simulink model "airTrackLab"  (R2021a)
settings: Solver=ode23t  StartTime=0.0  StopTime=30  FixedStep=0.02  MaxStep=0.01  RelTol=1e-3  AbsTol=1e-4  EnableMultiTasking=on
PostLoadFcn:
  | disp('default settings')
  | 
  | % Default starting positions
  | x0_cart1 = -0.2
  | x0_cart2 = 0.8
  | x0_gate1 = -0.4
  | x0_gate2 = 0.4
  | 
  | % How much damping the carts feel
  | dampingCoef = 0.01 % N/(m/s)
  | 
  | % Hanger damping
  | pulleyDamping = 0;
  | 
  | % Max measurement noise for the gates
  | noise_max = 0.01 % seconds
  | 
  | % How many time steps to show in the history
  | nHistory = 4
  | 
  | % Based on the provided STLs
  | cart_length = 0.15
  | 
  | subsystems = find_system(gcs,'BlockType','SubSystem');
  | p = Simulink.Mask.get(subsystems{1});
  | p.Parameters(1).Value = '-0.8';
  | p.Parameters(2).Value = '0';
  | p.Parameters(3).Value = '-0.4';
  | p.Parameters(4).Value = '0.4';
  | p.Parameters(5).Value = '0';
  | p.Parameters(6).Value = '0';
  | 
  | % Resize the model window
  | set(0,"Units","pixels")
  | sSize = get(0,"screensize");
  | set_param(gcs,'location',...
  |     [1,sSize(4)*0.01,round(sSize(3)/2),sSize(4)*0.96]);
  | 
  | % Reset the zoom
  | set_param(gcs, 'ZoomFactor','FitSystem')
undefined symbols (not defined in the file): X, Y, Z
libraries: sm_lib x104, simulink x12, nesl_utility x9
(part 1 of 3)
settings Model: EnablePacing=on  OrderedModelArguments=off  Creator=Rocksmithed  LastModifiedBy=Work
settings SolverCC: AutoScaleAbsTol=off  AlgebraicLoopSolver=TrustRegion
settings DataIOCC: LimitDataPoints=on  MaxDataPoints=10000
settings OptimizationCC: LifeSpan=inf
settings DebuggingCC: AllowSymbolicDim=off  SFUnexpectedBacktrackingDiag=warning  SFNoUnconditionalDefaultTransitionDiag=warning  SFExecutionAtInitializationDiag=none  SFMachineParentedDataDiag=warning  ArithmeticOperatorsInVariantConditions=warning
settings SFSimCC: SimUseLocalCustomCode=off  CustomCodeUndefinedFunction=UseInterfaceOnly
settings RTWCC: RTWUseLocalCustomCode=off
settings CodeAppCC: StateflowObjectComments=on
settings GRTTargetCC: TargetLangStandard=C89/C90 (ANSI)
settings ConfigComp: CovMetricSettings=dw  CovSaveCumulativeToWorkspaceVar=on  CovSaveSingleToWorkspaceVar=on  CovExternalEMLEnable=off  CovSFcnEnable=off
settings SimscapeCC: SimscapeLogType=all  SimscapeLogSimulationStatistics=on  SimscapeLogDataHistory=10000
settings ExplorerConfigSet: InternalSimMechanicsExplorerSettings="<ExplorerConfiguration><canonicalview>default</canonicalview><AnimationSetting><BasePlaybackSpeed>1.0</BasePlaybackSpeed><PlaybackSpeedFactor>1.0</PlaybackSpeedFactor></AnimationSetting><TilePanel><TileInfo><Tiles Columns=\"2\" Count=\"3\" Rows=\"2\"><Column Weight=\"0.8233\"/><Column Weight=\"0.1767\"/><Row Weight=\"0.2309\"/><Row Weight=\"0.7691\"/><Tile Height=\"1\" Width=\"2\" X=\"0\" Y=\"0\"/><Tile Height=\"1\" Width=\"1\" X=\"0\" Y=\"1\"/><Tile Height=\"1\" Width=\"1\" X=\"1\" Y=\"1\"/></Tiles></TileInfo><SceneInfo><SceneViewer><BGColor><R>1</R><G>1</G><B>1</B></BGColor><Camera><DoPerspective>off</DoPerspective><Position><X>0.018300882451578071</X><Y>-1.66502198042091809</Y><Z>0.155363278025413054</Z></Position><Center><X>0.018300882451578071</X><Y>9.39015043499580315e-09</Y><Z>0.155363278025413054</Z></Center><Up><X>0</X><Y>-0</Y><Z>1</Z></Up><ViewLimDist>1</ViewLimDist><YLim>0.387195273745834012</YLim><XLim>1.19850444036210479</XLim></Camera></SceneViewer><SceneViewer><BGColor><R>1</R><G>1</G><B>1</B></BGColor><Camera><DoPerspective>off</DoPerspective><Position><X>1.92657717822519481</X><Y>-0.555217561550410799</Y><Z>0.43190835445211162</Z></Position><Center><X>0.000630036713113105943</X><Y>-0.00292388052674194803</Y><Z>0.127558358447527082</Z></Center><Up><X>-0.139841397017632707</X><Y>0.0570909199469538109</Y><Z>0.988526686812130406</Z></Up><ViewLimDist>1</ViewLimDist><YLim>0.492618300070346571</YLim><XLim>0.372709129942266348</XLim></Camera></SceneViewer><SceneViewer><BGColor><R>1</R><G>1</G><B>1</B></BGColor><Camera><DoPerspective>off</DoPerspective><Position><X>1.02205702851478053</X><Y>-1.66502198042091809</Y><Z>-0.681352306661953344</Z></Position><Center><X>1.02205702851478053</X><Y>8.09732611517510747e-09</Y><Z>-0.681352306661953344</Z></Center><Up><X>0</X><Y>-0</Y><Z>1</Z></Up><ViewLimDist>1</ViewLimDist><YLim>1.06828991799173401</YLim><XLim>0.17113382181420983</XLim></Camera></SceneViewer></SceneInfo></TilePanel><MechEditorPanel><Cameras><Camera><Id>Camera1</Id><Value><Name>Camera1</Name><NativeCamera><PositionKeyframeSet><Keyframe><Time>30</Time><Value><X>-0.06353733975693017</X><Y>-1.5549717096079039</Y><Z>0.94456927641812571</Z></Value></Keyframe></PositionKeyframeSet><CenterKeyframeSet><Keyframe><Time>30</Time><Value><X>-0.014695794825631658</X><Y>-0.017005502884078094</Y><Z>0.19960924384738066</Z></Value></Keyframe></CenterKeyframeSet><UpVectorKeyframeSet><Keyframe><Time>30</Time><Value><X>-0.0033381063490633966</X><Y>0.43601551279510337</Y><Z>0.89993295841858445</Z></Value></Keyframe></UpVectorKeyframeSet></NativeCamera></Value></Camera></Cameras><GfxPanelCameraMap/><VideoCreator><PlaybackSpeedRatio>1.0</PlaybackSpeedRatio><FrameRate>30</FrameRate><VideoFormat>Motion JPEG AVI</VideoFormat><FrameSize>auto</FrameSize></VideoCreator></MechEditorPanel></ExplorerConfiguration>"

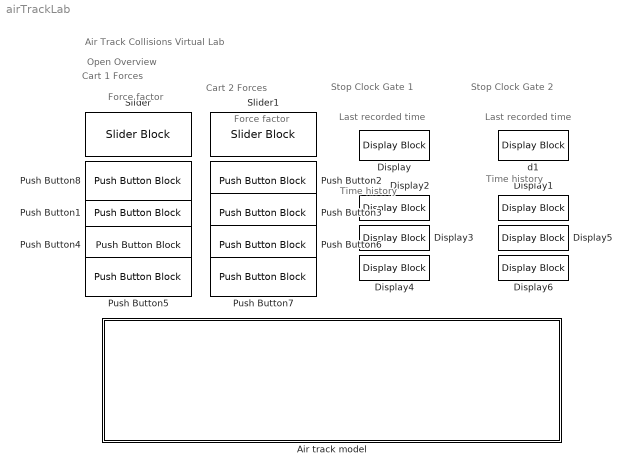
== system airTrackLab ==
  note: Air Track Collisions Virtual Lab
  note: Open Overview
  note: Force factor
  note: Stop Clock Gate 2
  note: Cart 1 Forces
  note: Cart 2 Forces
  note: Stop Clock Gate 1
  note: Force factor
  note: Last recorded time
  note: Time history
  note: Last recorded time
  note: Time history
  Air track model : Subsystem  InitFcn=|  mask{popup_collisionType=Elastic, x0_cart1=-0.8, x0_gate1=-0.4, x0_cart2=0, x0_gate2=0.4, popup_extraMassC1=0 plates (0 g), popup_extraMassC2=0 plates (0 g), popup_hangingMass=0 plates (0 g)}
      | if(x0_cart1 > x0_cart2)
      | 	error('Set cart 2 to be on the + side of cart 1')
      |    x0_cart1 = -0.75;
      |    x0_cart2 = 0.75;
      | end
      mask prompts: popup_collisionType "Collisions"; x0_cart1 "Cart 1 x0 [m] (must be left of Cart 2)"; x0_gate1 "Gate 1 x [m]"; x0_cart2 "Cart 2 x0 [m] (must be right of Cart 1)"; x0_gate2 "Gate 2 x [m]"; popup_extraMassC1 "Cart 1"; popup_extraMassC2 "Cart 2"; popup_hangingMass "Hanging"
      mask init:
      | set_param([gcb '/Contact Force'],'LabelModeActiveChoice',get_param(gcb,'popup_collisionType'));
      | switch(get_param(gcb,'popup_extraMassC1'))
      |     case '0 plates (0 g)', vntstrC1 = 'None';
      |     case '1 plate (100 g)', vntstrC1 = 'Plates_1';
      |     case '2 plates (200 g)',vntstrC1 = 'Plates_2';
      |     case '3 plates (300 g)',vntstrC1 = 'Plates_3';
      | end
      | set_param([gcb '/Mass Cart 1'],'LabelModeActiveChoice',vntstrC1);
      | switch(get_param(gcb,'popup_extraMassC2'))
      |     case '0 plates (0 g)', vntstrC2 = 'None';
      |     case '1 plate (100 g)', vntstrC2 = 'Plates_1';
      |     case '2 plates (200 g)',vntstrC2 = 'Plates_2';
      |     case '3 plates (300 g)',vntstrC2 = 'Plates_3';
      | end
      | set_param([gcb '/Mass Cart 2'],'LabelModeActiveChoice',vntstrC2);
      | 
      | switch(get_param(gcb,'popup_hangingMass'))
      |     case '0 plates (0 g)', vntstrH = 'None'; 
      |     case '1 plate (100 g)', vntstrH = 'Plates_1';
      |     case '2 plates (200 g)',vntstrH = 'Plates_2';
      |     case '3 plates (300 g)',vntstrH = 'Plates_3';
      | end
      | if(strcmp(vntstrH,'None'))
      | set_param([gcb '/Load'],'LabelModeActiveChoice','None');
      | else
      | set_param([gcb '/Load'],'LabelModeActiveChoice','Hanging_Mass');
      | set_param([gcb '/Load/Hanging Mass/Mass'],'LabelModeActiveChoice',vntstrH);
      | end
      mask TypeOptions popup_collisionType: Elastic | Inelastic
      mask Callback x0_cart1:
      | maskObj = Simulink.Mask.get(gcb);
      | x0c1_h = maskObj.getParameter('x0_cart1');
      | x0c2_h = maskObj.getParameter('x0_cart2');
      | if(str2num(x0c2_h.Value)<=(str2num(x0c1_h.Value)+0.165))
      |    x0c2_h.Value=num2str(round(str2num(x0c1_h.Value)+0.165+0.0005,3));
      |    %x0c2_h.Value = num2str(0);
      | end
      | x0c2_h.Range=[str2num(x0c1_h.Value)+0.165 0.8];
      | 
      | %clear maskObj
      mask Callback x0_cart2:
      | maskObj = Simulink.Mask.get(gcb);
      | x0c1_h = maskObj.getParameter('x0_cart1');
      | x0c2_h = maskObj.getParameter('x0_cart2');
      | if(str2num(x0c1_h.Value)>=(str2num(x0c2_h.Value)-0.165))
      |    x0c2_h.Value=num2str(round(str2num(x0c2_h.Value)-0.165-0.0005,3));
      |    %x0c2_h.Value = num2str(0);
      | end
      | x0c1_h.Range=[-0.8 str2num(x0c2_h.Value)-0.165];
      mask TypeOptions popup_extraMassC1: 0 plates (0 g) | 1 plate (100 g) | 2 plates (200 g) | 3 plates (300 g)
      mask TypeOptions popup_extraMassC2: 0 plates (0 g) | 1 plate (100 g) | 2 plates (200 g) | 3 plates (300 g)
      mask TypeOptions popup_hangingMass: 0 plates (0 g) | 1 plate (100 g) | 2 plates (200 g) | 3 plates (300 g)
      mask DialogControl Container7 Prompt: Experiments
      mask DialogControl push_default Prompt: Default Setup
      mask DialogControl push_default Callback:
      | maskObj = Simulink.Mask.get(gcb);
      | x0c1_h = maskObj.getParameter('x0_cart1');
      | x0c1_h.Value = '-0.8';
      | x0c2_h = maskObj.getParameter('x0_cart2');
      | x0c2_h.Value = '0';
      | 
      | x0c1_h.Range = [-0.8 -0.165];
      | x0c2_h.Range = [-0.635 0.8];
      | 
      | x0g1_h = maskObj.getParameter('x0_gate1');
      | x0g1_h.Value = '-0.4';
      | x0g2_h = maskObj.getParameter('x0_gate2');
      | x0g2_h.Value = '0.4';
      | pmc1_h = maskObj.getParameter('popup_extraMassC1');
      | pmc1_h.Value = '0 plates (0 g)';
      | pmc2_h = maskObj.getParameter('popup_extraMassC2');
      | pmc2_h.Value = '0 plates (0 g)';
      | phm_h = maskObj.getParameter('popup_hangingMass');
      | phm_h.Value = '0 plates (0 g)';
      | pct_h = maskObj.getParameter('popup_collisionType');
      | pct_h.Value = 'Elastic';
      | 
      | clear maskObj
      mask DialogControl push_default_copy Prompt: 1. Elastic
      mask DialogControl push_default_copy Callback:
      | maskObj = Simulink.Mask.get(gcb);
      | x0c1_h = maskObj.getParameter('x0_cart1');
      | x0c1_h.Value = '-0.8';
      | x0c2_h = maskObj.getParameter('x0_cart2');
      | x0c2_h.Value = '0';
      | 
      | x0c1_h.Range = [-0.8 -0.165];
      | x0c2_h.Range = [-0.635 0.8];
      | 
      | x0g1_h = maskObj.getParameter('x0_gate1');
      | x0g1_h.Value = '-0.4';
      | x0g2_h = maskObj.getParameter('x0_gate2');
      | x0g2_h.Value = '0.4';
      | pmc1_h = maskObj.getParameter('popup_extraMassC1');
      | pmc1_h.Value = '0 plates (0 g)';
      | pmc2_h = maskObj.getParameter('popup_extraMassC2');
      | pmc2_h.Value = '0 plates (0 g)';
      | phm_h = maskObj.getParameter('popup_hangingMass');
      | phm_h.Value = '0 plates (0 g)';
      | pct_h = maskObj.getParameter('popup_collisionType');
      | pct_h.Value = 'Elastic';
      | 
      | clear maskObj
      mask DialogControl push_default_copy_copy Prompt: 2. Inelastic
      mask DialogControl push_default_copy_copy Callback:
      | maskObj = Simulink.Mask.get(gcb);
      | x0c1_h = maskObj.getParameter('x0_cart1');
      | x0c1_h.Value = '-0.8';
      | x0c2_h = maskObj.getParameter('x0_cart2');
      | x0c2_h.Value = '0';
      | 
      | x0c1_h.Range = [-0.8 -0.165];
      | x0c2_h.Range = [-0.635 0.8];
      | 
      | x0g1_h = maskObj.getParameter('x0_gate1');
      | x0g1_h.Value = '-0.4';
      | x0g2_h = maskObj.getParameter('x0_gate2');
      | x0g2_h.Value = '0.4';
      | pmc1_h = maskObj.getParameter('popup_extraMassC1');
      | pmc1_h.Value = '3 plates (300 g)';
      | pmc2_h = maskObj.getParameter('popup_extraMassC2');
      | pmc2_h.Value = '0 plates (0 g)';
      | phm_h = maskObj.getParameter('popup_hangingMass');
      | phm_h.Value = '0 plates (0 g)';
      | pct_h = maskObj.getParameter('popup_collisionType');
      | pct_h.Value = 'Inelastic';
      | 
      | clear maskObj
      mask DialogControl push_default_copy_copy_copy Prompt: 3. Energy
      mask DialogControl push_default_copy_copy_copy Callback:
      | maskObj = Simulink.Mask.get(gcb);
      | x0c1_h = maskObj.getParameter('x0_cart1');
      | x0c1_h.Value = '-0.8';
      | x0c2_h = maskObj.getParameter('x0_cart2');
      | x0c2_h.Value = '0';
      | 
      | x0c1_h.Range = [-0.8 -0.165];
      | x0c2_h.Range = [-0.635 0.8];
      | 
      | x0g1_h = maskObj.getParameter('x0_gate1');
      | x0g1_h.Value = '0.3';
      | x0g2_h = maskObj.getParameter('x0_gate2');
      | x0g2_h.Value = '0.6';
      | pmc1_h = maskObj.getParameter('popup_extraMassC1');
      | pmc1_h.Value = '0 plates (0 g)';
      | pmc2_h = maskObj.getParameter('popup_extraMassC2');
      | pmc2_h.Value = '2 plates (200 g)';
      | phm_h = maskObj.getParameter('popup_hangingMass');
      | phm_h.Value = '1 plate (100 g)';
      | pct_h = maskObj.getParameter('popup_collisionType');
      | pct_h.Value = 'Elastic';
      | 
      | clear maskObj
      mask DialogControl Container10 Prompt: Extra Mass
      mask Display:
      | image('airTrackMask.png','center');
      | text(0.12, 0.79, 'Cart 1', 'horizontalAlignment', 'center')
      | text(0.86, 0.79, 'Cart 2', 'horizontalAlignment', 'center')
      | 
      | text(0.32, 0.87, 'Gate 1', 'horizontalAlignment', 'center')
      | text(0.67, 0.87, 'Gate 2', 'horizontalAlignment', 'center')
      | 
      | text(0.5, 0.1, 'Double-click here to set starting positions and weights', 'horizontalAlignment', 'center')
      | 
      | text(0.91, 0.17, '+ direction', 'horizontalAlignment', 'center')
  Display{,1..4} (5 alike) : DisplayBlock  LabelPosition=Hide  Format=short  Transparency=1
  Display5 : DisplayBlock  LabelPosition=Hide  Format=short  Transparency=1  Layout=Fill available space
  Display6 : DisplayBlock  LabelPosition=Hide  Format=short  Transparency=1  Layout=Fill available space
  Push Button1 : PushButtonBlock  ButtonText=Apply force -x
  Push Button2 : PushButtonBlock  ButtonText=Apply force +x
  Push Button3 : PushButtonBlock  ButtonText=Apply force -x
  Push Button4 : PushButtonBlock  ButtonText=Pulse +x (0.1 sec)
  Push Button5 : PushButtonBlock  ButtonText=Pulse -x (0.1 sec)  OnValue=-1
  Push Button6 : PushButtonBlock  ButtonText=Pulse +x (0.1 sec)
  Push Button7 : PushButtonBlock  ButtonText=Pulse -x (0.1 sec)  OnValue=-1
  Push Button8 : PushButtonBlock  ButtonText=Apply force +x
  Slider : SliderBlock  LabelPosition=Hide  ScaleMax=1  TickInterval=0.25
  Slider1 : SliderBlock  LabelPosition=Hide  ScaleMax=1  TickInterval=0.25
  d1 : DisplayBlock  LabelPosition=Hide  Format=short  Transparency=1  Layout=Fill available space

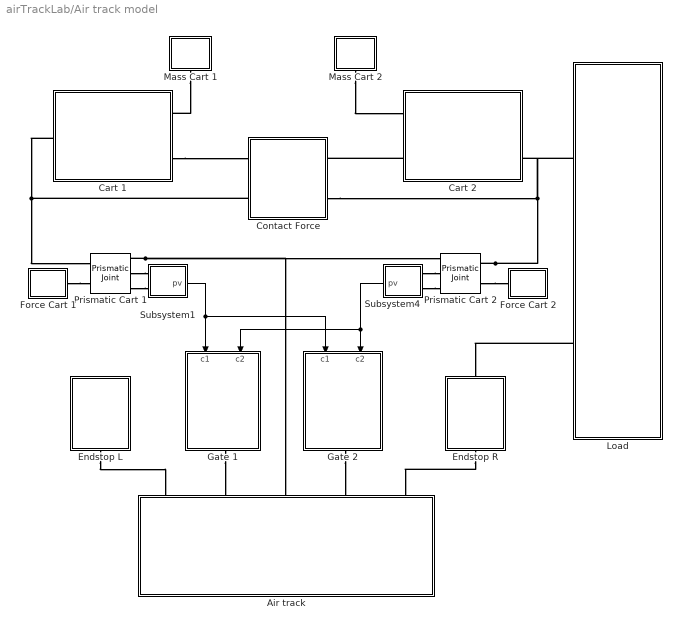
== system airTrackLab/Air track model ==
  Air track : Subsystem
      settings: PortSchema="{\"entries\":[{\"content\":{\"sides\":[{\"content\":{\"connectorIds\":[]},\"type\":\"ConnectorPlacement.EquallySpacedRectSide\",\"uuid\":\"090b3a62-51f7-462c-98c5-a584c300c54a\"},{\"content\":{\"connectorIds\":[],\"side\":\"RIGHT\"},\"type\":\"ConnectorPlacement.EquallySpacedRectSide\",\"uuid\":\"a4dd45ef-3830-4d80-a6d2-012ce92ee2ce\"},{\"content\":{\"connectorIds\":[],\"side\":\"TOP\"},\"type\":\"ConnectorPlacement.EquallySpacedRectSide\",\"uuid\":\"395c260b-744a-480a-9e83-719a01711115\"},{\"content\":{\"connectorIds\":[\"RConn1\",\"RConn2\",\"RConn3\",\"RConn4\",\"RConn5\"],\"side\":\"BOTTOM\"},\"type\":\"ConnectorPlacement.EquallySpacedRectSide\",\"uuid\":\"a18b275a-4662-4f32-9408-960fb193559a\"}]},\"type\":\"ConnectorPlacement.EquallySpacedConnector\",\"uuid\":\"2f11ba3c-3a56-4e43-8d79-c5dc35ee6124\"}],\"packageUris\":[\"http://schema.mathworks.com/mf0/Connector/R2020b\"],\"version\":\"1.0\"}"
      mask Display: image('airTrack.png');
  Cart 1 : Subsystem
      mask Display: image('cart.png');
  Cart 2 : Subsystem
      mask Display: image('cart.png');
  Contact Force : Subsystem  Variant=on  VariantControlMode=label  VariantControl=Choice  LabelModeActiveChoice=Elastic
  Endstop L : Subsystem
      mask Display: image('stop.png');
  Endstop R : Subsystem
      mask Display: image('stop.png');
  Force Cart 1 : Subsystem
  Force Cart 2 : Subsystem
  Gate 1 : Subsystem
      mask Display: image('gate1.png');
  Gate 2 : Subsystem
      mask Display: image('gate2.png');
  Load : Subsystem  Variant=on  VariantControlMode=label  VariantControl=Choice  LabelModeActiveChoice=None
      settings: AttributesFormatString=%<LabelModeActiveChoice>
  Mass Cart 1 : Subsystem  Variant=on  VariantControlMode=label  VariantControl=Choice  LabelModeActiveChoice=None
      settings: AttributesFormatString=%<LabelModeActiveChoice>
  Mass Cart 2 : Subsystem  Variant=on  VariantControlMode=label  VariantControl=Choice  LabelModeActiveChoice=None
      settings: AttributesFormatString=%<LabelModeActiveChoice>
  Prismatic Cart 1 : sm_lib/Joints/Prismatic Joint  JointMode=Normal  SenseConstraintForce=off  SenseConstraintForceX=off  SenseConstraintForceY=off  SenseConstraintForceZ=off  SenseConstraintTorque=off  SenseConstraintTorqueX=off  SenseConstraintTorqueY=off  SenseConstraintTorqueZ=off  SenseTotalForce=off  SenseTotalForceX=off  SenseTotalForceY=off  SenseTotalForceZ=off  SenseTotalTorque=off  SenseTotalTorqueX=off  SenseTotalTorqueY=off  SenseTotalTorqueZ=off  CompositeWrenchDir=FollowerOnBase  CompositeWrenchFrame=BaseFrame  EquilibriumPosition=0  EquilibriumPositionUnits=m  SpringStiffness=0  SpringStiffnessUnits=N/m  DampingCoefficient=dampingCoef  DampingCoefficientUnits=N/(m/s)  TorqueActuationMode=InputTorque  MotionActuationMode=ComputedMotion  SensePosition=on  SenseVelocity=on  SenseAcceleration=off  SenseTorqueForce=off  SenseLowerLimitTorqueForce=off  SenseUpperLimitTorqueForce=off  LowerLimitSpecify=on  LowerLimitBound=-0.9  LowerLimitBoundUnits=m  LowerLimitStiffness=1e9  LowerLimitStiffnessUnits=N/m  LowerLimitDamping=0.1  LowerLimitDampingUnits=N/(m/s)  LowerLimitTransitionRegionWidth=1e-4  LowerLimitTransitionRegionWidthUnits=m  UpperLimitSpecify=on  UpperLimitBound=0.9  UpperLimitBoundUnits=m  UpperLimitStiffness=1e9  UpperLimitStiffnessUnits=N/m  UpperLimitDamping=0.1  UpperLimitDampingUnits=N/(m/s)  UpperLimitTransitionRegionWidth=1e-4  UpperLimitTransitionRegionWidthUnits=m  PositionTargetSpecify=on  PositionTargetPriority=High  PositionTargetValue=x0_cart1  PositionTargetValueUnits=m  VelocityTargetSpecify=off  VelocityTargetPriority=High  VelocityTargetValue=0.5  VelocityTargetValueUnits=m/s
  Prismatic Cart 2 : sm_lib/Joints/Prismatic Joint  JointMode=Normal  SenseConstraintForce=off  SenseConstraintForceX=off  SenseConstraintForceY=off  SenseConstraintForceZ=off  SenseConstraintTorque=off  SenseConstraintTorqueX=off  SenseConstraintTorqueY=off  SenseConstraintTorqueZ=off  SenseTotalForce=off  SenseTotalForceX=off  SenseTotalForceY=off  SenseTotalForceZ=off  SenseTotalTorque=off  SenseTotalTorqueX=off  SenseTotalTorqueY=off  SenseTotalTorqueZ=off  CompositeWrenchDir=FollowerOnBase  CompositeWrenchFrame=BaseFrame  EquilibriumPosition=0  EquilibriumPositionUnits=m  SpringStiffness=0  SpringStiffnessUnits=N/m  DampingCoefficient=dampingCoef  DampingCoefficientUnits=N/(m/s)  TorqueActuationMode=InputTorque  MotionActuationMode=ComputedMotion  SensePosition=on  SenseVelocity=on  SenseAcceleration=off  SenseTorqueForce=off  SenseLowerLimitTorqueForce=off  SenseUpperLimitTorqueForce=off  LowerLimitSpecify=on  LowerLimitBound=-0.9  LowerLimitBoundUnits=m  LowerLimitStiffness=1e9  LowerLimitStiffnessUnits=N/m  LowerLimitDamping=0.1  LowerLimitDampingUnits=N/(m/s)  LowerLimitTransitionRegionWidth=1e-4  LowerLimitTransitionRegionWidthUnits=m  UpperLimitSpecify=on  UpperLimitBound=0.9  UpperLimitBoundUnits=m  UpperLimitStiffness=1e9  UpperLimitStiffnessUnits=N/m  UpperLimitDamping=0.1  UpperLimitDampingUnits=N/(m/s)  UpperLimitTransitionRegionWidth=1e-4  UpperLimitTransitionRegionWidthUnits=m  PositionTargetSpecify=on  PositionTargetPriority=High  PositionTargetValue=x0_cart2  PositionTargetValueUnits=m  VelocityTargetSpecify=off  VelocityTargetPriority=High  VelocityTargetValue=0.5  VelocityTargetValueUnits=m/s
  Subsystem1 : Subsystem
  Subsystem4 : Subsystem
  wires:
  Subsystem1/1(pv) -> Gate 2/1(c1), Gate 1/1(c1)
  Subsystem4/1(pv) -> Gate 1/2(c2), Gate 2/2(c2)
  connections:
  Gate 2/RConn1 -- Air track/RConn2
  Gate 1/RConn1 -- Air track/RConn4
  Endstop L/RConn1 -- Air track/RConn5
  Endstop R/RConn1 -- Air track/RConn1
  Prismatic Cart 1/RConn3 -- Subsystem1/LConn2
  Prismatic Cart 1/RConn2 -- Subsystem1/LConn1
  Force Cart 1/RConn1 -- Prismatic Cart 1/LConn2
  Cart 1/RConn2 -- Contact Force/LConn1
  Subsystem4/LConn2 -- Prismatic Cart 2/RConn3
  Subsystem4/LConn1 -- Prismatic Cart 2/RConn2
  Prismatic Cart 2/LConn2 -- Force Cart 2/RConn1
  Prismatic Cart 1/RConn1 -- Prismatic Cart 2/RConn1 -- Air track/RConn3
  Mass Cart 2/RConn1 -- Cart 2/LConn1
  Cart 2/LConn2 -- Contact Force/RConn1
  Cart 1/LConn1 -- Prismatic Cart 1/LConn1 -- Contact Force/LConn2
  Prismatic Cart 2/LConn1 -- Contact Force/RConn2 -- Load/LConn1 -- Cart 2/RConn2
  Load/LConn2 -- Endstop R/LConn1
  Mass Cart 1/RConn1 -- Cart 1/RConn1

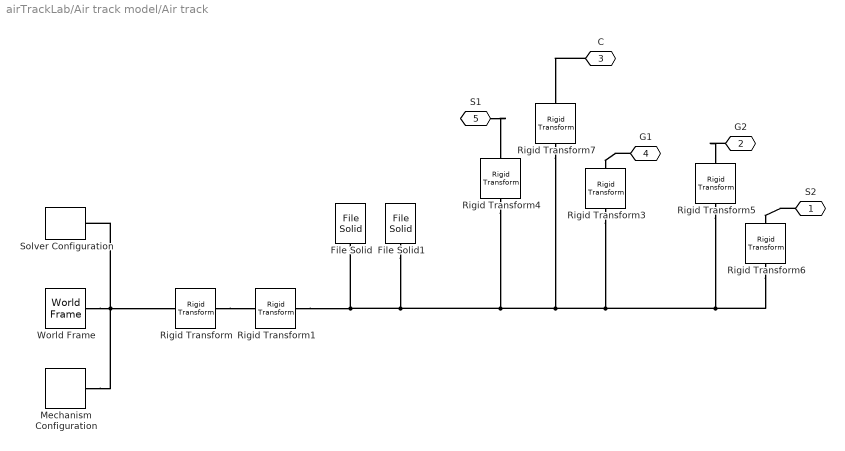
== system airTrackLab/Air track model/Air track ==
  File Solid : sm_lib/Body Elements/File Solid  ExtGeomFileName=airTrack.stl  UnitType=Custom  ExtGeomFileUnits=mm  StepReaderType=HEX  ExportConvexHullGeometry=off  InertiaType=CalculateFromGeometry  Mass=1  MassUnits=kg  CenterOfMass=[0 0 0]  CenterOfMassUnits=m  MomentsOfInertia=[1 1 1]  MomentsOfInertiaUnits=kg*m^2  ProductsOfInertia=[0 0 0]  ProductsOfInertiaUnits=kg*m^2  BasedOnType=Density  Density=1000  DensityUnits=kg/m^3  DoExposeReferenceFrame=on  SerializedFrames=<Frames><Frame><Id>Frame1</Id><Value><Name>F1</Name><Origin><Source>CenterOfMassFrame</Source><FeatureName></FeatureName></Origin><PrimaryAxis><DefinedDirection>+X</DefinedDirection><Source>ReferenceFrame</Source><SourceDirection>+Z</SourceDirection><FeatureName></FeatureName></PrimaryAxis><SecondaryAxis><DefinedDirection>+Y</DefinedDirection><Source>ReferenceFrame</Source><SourceDirection>+X</SourceDirection><FeatureName></FeatureName></SecondaryAxis></Value></Frame></Frames>  GraphicType=FromGeometry  MarkerShape=Sphere  MarkerSize=10  GraphicVisPropType=AdvancedVisualProperties  GraphicDiffuseColor=[0.8 0.8 0.81]  GraphicSpecularColor=[0.7 0.7 0.7 1]  GraphicAmbientColor=[0.05 0.05 0.05 1]  GraphicEmissiveColor=[0.05 0.05 0.05 1.0]  GraphicShininess=15  GraphicOpacity=1.0
  File Solid1 : sm_lib/Body Elements/File Solid  ExtGeomFileName=ruler.stl  UnitType=Custom  ExtGeomFileUnits=mm  StepReaderType=HEX  ExportConvexHullGeometry=off  InertiaType=CalculateFromGeometry  Mass=1  MassUnits=kg  CenterOfMass=[0 0 0]  CenterOfMassUnits=m  MomentsOfInertia=[1 1 1]  MomentsOfInertiaUnits=kg*m^2  ProductsOfInertia=[0 0 0]  ProductsOfInertiaUnits=kg*m^2  BasedOnType=Density  Density=1000  DensityUnits=kg/m^3  DoExposeReferenceFrame=on  SerializedFrames=<Frames><Frame><Id>Frame1</Id><Value><Name>F1</Name><Origin><Source>CenterOfMassFrame</Source><FeatureName></FeatureName></Origin><PrimaryAxis><DefinedDirection>+X</DefinedDirection><Source>ReferenceFrame</Source><SourceDirection>+Z</SourceDirection><FeatureName></FeatureName></PrimaryAxis><SecondaryAxis><DefinedDirection>+Y</DefinedDirection><Source>ReferenceFrame</Source><SourceDirection>+X</SourceDirection><FeatureName></FeatureName></SecondaryAxis></Value></Frame></Frames>  GraphicType=FromGeometry  MarkerShape=Sphere  MarkerSize=10  GraphicVisPropType=AdvancedVisualProperties  GraphicDiffuseColor="[0.9882    0.9176    0.0902]"  GraphicSpecularColor="[0.5882    0.5176    0.0902 1]"  GraphicAmbientColor=[0.05 0.05 0.05 1]  GraphicEmissiveColor=[0.15 0.15 0.1 1.0]  GraphicShininess=20  GraphicOpacity=1.0
  Mechanism Configuration : sm_lib/Utilities/Mechanism Configuration  UniformGravity=Constant  GravityVector=[0 0 -9.80665]  GravityVectorUnits=m/s^2  GravityUnits=m/s^2  LinearizationDelta=0.001  JointModeTransitionNonlinearIterations=2
  Rigid Transform : sm_lib/Frames and Transforms/Rigid Transform  TranslationMethod=Cartesian  TranslationStandardOffset=0  TranslationLengthUnit=m  TranslationStandardAxis=+Z  TranslationCartesianOffset=[0 0 0.02]  TranslationROffset=0  TranslationROffsetUnits=m  TranslationZOffset=0  TranslationZOffsetUnits=m  TranslationThetaOffset=0  TranslationThetaOffsetUnits=deg  RotationMethod=StandardAxis  RotationAngleUnits=deg  RotationStandardAxis=+X  RotationAngle=90  RotationArbitraryAxis=[0 0 1]  FollAlignAxisA=+X  BaseAlignAxisA=+Y  FollAlignAxisB=+Y  BaseAlignAxisB=+Z  RotationSequenceAxes=FollowerAxes  RotationSequence=XYX  RotationSequenceAngles=[0 0 0]  RotationSequenceAnglesUnits=deg  RotationMatrix=[1 0 0; 0 1 0; 0 0 1]
  Rigid Transform1 : sm_lib/Frames and Transforms/Rigid Transform  TranslationMethod=None  TranslationStandardOffset=0  TranslationLengthUnit=m  TranslationStandardAxis=+Z  TranslationCartesianOffset=[0 0 0]  TranslationROffset=0  TranslationROffsetUnits=m  TranslationZOffset=0  TranslationZOffsetUnits=m  TranslationThetaOffset=0  TranslationThetaOffsetUnits=deg  RotationMethod=StandardAxis  RotationAngleUnits=deg  RotationStandardAxis=+Y  RotationAngle=180  RotationArbitraryAxis=[0 0 1]  FollAlignAxisA=+X  BaseAlignAxisA=+Y  FollAlignAxisB=+Y  BaseAlignAxisB=+Z  RotationSequenceAxes=FollowerAxes  RotationSequence=XYX  RotationSequenceAngles=[0 0 0]  RotationSequenceAnglesUnits=deg  RotationMatrix=[1 0 0; 0 1 0; 0 0 1]
  Rigid Transform3 : sm_lib/Frames and Transforms/Rigid Transform  TranslationMethod=Cartesian  TranslationStandardOffset=x0_cart2  TranslationLengthUnit=m  TranslationStandardAxis=+X  TranslationCartesianOffset=[-x0_gate1 0 0 ]  TranslationROffset=0  TranslationROffsetUnits=m  TranslationZOffset=0  TranslationZOffsetUnits=m  TranslationThetaOffset=0  TranslationThetaOffsetUnits=deg  RotationMethod=None  RotationAngleUnits=deg  RotationStandardAxis=+Z  RotationAngle=0.0  RotationArbitraryAxis=[0 0 1]  FollAlignAxisA=+X  BaseAlignAxisA=+Y  FollAlignAxisB=+Y  BaseAlignAxisB=+Z  RotationSequenceAxes=FollowerAxes  RotationSequence=XYX  RotationSequenceAngles=[0 0 0]  RotationSequenceAnglesUnits=deg  RotationMatrix=[1 0 0; 0 1 0; 0 0 1]
  Rigid Transform4 : sm_lib/Frames and Transforms/Rigid Transform  TranslationMethod=StandardAxis  TranslationStandardOffset=1.985  TranslationLengthUnit=m  TranslationStandardAxis=+X  TranslationCartesianOffset=[0 0 0]  TranslationROffset=0  TranslationROffsetUnits=m  TranslationZOffset=0  TranslationZOffsetUnits=m  TranslationThetaOffset=0  TranslationThetaOffsetUnits=deg  RotationMethod=None  RotationAngleUnits=deg  RotationStandardAxis=+Z  RotationAngle=0.0  RotationArbitraryAxis=[0 0 1]  FollAlignAxisA=+X  BaseAlignAxisA=+Y  FollAlignAxisB=+Y  BaseAlignAxisB=+Z  RotationSequenceAxes=FollowerAxes  RotationSequence=XYX  RotationSequenceAngles=[0 0 0]  RotationSequenceAnglesUnits=deg  RotationMatrix=[1 0 0; 0 1 0; 0 0 1]
  Rigid Transform5 : sm_lib/Frames and Transforms/Rigid Transform  TranslationMethod=Cartesian  TranslationStandardOffset=x0_cart2  TranslationLengthUnit=m  TranslationStandardAxis=+X  TranslationCartesianOffset=[-x0_gate2 0 0]  TranslationROffset=0  TranslationROffsetUnits=m  TranslationZOffset=0  TranslationZOffsetUnits=m  TranslationThetaOffset=0  TranslationThetaOffsetUnits=deg  RotationMethod=None  RotationAngleUnits=deg  RotationStandardAxis=+Z  RotationAngle=0.0  RotationArbitraryAxis=[0 0 1]  FollAlignAxisA=+X  BaseAlignAxisA=+Y  FollAlignAxisB=+Y  BaseAlignAxisB=+Z  RotationSequenceAxes=FollowerAxes  RotationSequence=XYX  RotationSequenceAngles=[0 0 0]  RotationSequenceAnglesUnits=deg  RotationMatrix=[1 0 0; 0 1 0; 0 0 1]
  Rigid Transform6 : sm_lib/Frames and Transforms/Rigid Transform  TranslationMethod=Cartesian  TranslationStandardOffset=0  TranslationLengthUnit=m  TranslationStandardAxis=+X  TranslationCartesianOffset=[0 0 0]  TranslationROffset=0  TranslationROffsetUnits=m  TranslationZOffset=0  TranslationZOffsetUnits=m  TranslationThetaOffset=0  TranslationThetaOffsetUnits=deg  RotationMethod=None  RotationAngleUnits=deg  RotationStandardAxis=+Z  RotationAngle=0.0  RotationArbitraryAxis=[0 0 1]  FollAlignAxisA=+X  BaseAlignAxisA=+Y  FollAlignAxisB=+Y  BaseAlignAxisB=+Z  RotationSequenceAxes=FollowerAxes  RotationSequence=XYX  RotationSequenceAngles=[0 0 0]  RotationSequenceAnglesUnits=deg  RotationMatrix=[1 0 0; 0 1 0; 0 0 1]
  Rigid Transform7 : sm_lib/Frames and Transforms/Rigid Transform  TranslationMethod=None  TranslationStandardOffset=0  TranslationLengthUnit=m  TranslationStandardAxis=+Z  TranslationCartesianOffset=[0 0 0]  TranslationROffset=0  TranslationROffsetUnits=m  TranslationZOffset=0  TranslationZOffsetUnits=m  TranslationThetaOffset=0  TranslationThetaOffsetUnits=deg  RotationMethod=StandardAxis  RotationAngleUnits=deg  RotationStandardAxis=+Y  RotationAngle=-90  RotationArbitraryAxis=[0 0 1]  FollAlignAxisA=+X  BaseAlignAxisA=+Y  FollAlignAxisB=+Y  BaseAlignAxisB=+Z  RotationSequenceAxes=FollowerAxes  RotationSequence=XYX  RotationSequenceAngles=[0 0 0]  RotationSequenceAnglesUnits=deg  RotationMatrix=[1 0 0; 0 1 0; 0 0 1]
  Solver Configuration : nesl_utility/Solver Configuration  PhysicalDomain=network_engine_domain  SubClassName=solver  LeftPortType=input  RightPortType=generic  Tones=[]  Harmonics=[]  SimulateNoise=off  Profile=off  UseLocalSampling=off  EnableSwitchedLinearOptims=on  FrequencyDomain=off  UseCCode=off  RelTol=0.001  AbsTol=1e-06  MinStep=1e-09  ToWorkspace=off  RevertToSquareIcSolve=off  NumHomotopyIterations=100  PhasorMode=off  PhasorModeNumHarmonics=1  DoDC=off  ResidualTolerance=1e-09  UseLocalSolver=off  LocalSolverChoice=NE_BACKWARD_EULER_ADVANCER  LocalSolverSampleTime=0.001  DoFixedCost=off  MaxNonlinIter=3  MaxModeIter=2  ComputeImpulses=off  ImpulseIterations=2  LinearAlgebra=Sparse  EquationFormulation=NE_TIME_EF  DelaysMemoryBudget=1024  AutomaticFiltering=on  FilteringTimeConstant=0.001  PartitionStorageMethod=AS_NEEDED  PartitionMemoryBudget=1024  PartitionMethod=FAST
      settings: SourceProductBaseCode=PW,SS
  World Frame : sm_lib/Frames and Transforms/World Frame
  S2 : PMIOPort  Side=Right
  G2 : PMIOPort  Port=2  Side=Right
  C : PMIOPort  Port=3  Side=Right
  G1 : PMIOPort  Port=4  Side=Right
  S1 : PMIOPort  Port=5  Side=Right
  connections:
  File Solid/RConn1 -- Rigid Transform7/RConn1 -- Rigid Transform6/LConn1 -- Rigid Transform5/LConn1 -- Rigid Transform3/LConn1 -- Rigid Transform4/LConn1 -- File Solid1/RConn1 -- Rigid Transform1/RConn1
  Rigid Transform/RConn1 -- Rigid Transform1/LConn1
  Mechanism Configuration/RConn1 -- Solver Configuration/RConn1 -- Rigid Transform/LConn1 -- World Frame/RConn1
  G1/RConn1 -- Rigid Transform3/RConn1
  S1/RConn1 -- Rigid Transform4/RConn1
  G2/RConn1 -- Rigid Transform5/RConn1
  S2/RConn1 -- Rigid Transform6/RConn1
  C/RConn1 -- Rigid Transform7/LConn1

== system airTrackLab/Air track model/Cart 1 ==
  note: The cart has a mass of 180 grams and a length of 15cm
  File Solid2 : sm_lib/Body Elements/File Solid  ExtGeomFileName=cart.stl  UnitType=Custom  ExtGeomFileUnits=mm  StepReaderType=HEX  ExportConvexHullGeometry=off  InertiaType=PointMass  Mass=180  MassUnits=g  CenterOfMass=[0 0 0]  CenterOfMassUnits=m  MomentsOfInertia=[1 1 1]  MomentsOfInertiaUnits=kg*m^2  ProductsOfInertia=[0 0 0]  ProductsOfInertiaUnits=kg*m^2  BasedOnType=Density  Density=1000  DensityUnits=kg/m^3  DoExposeReferenceFrame=on  SerializedFrames=<Frames><Frame><Id>Frame1</Id><Value><Name>F1</Name><Origin><Source>CenterOfMassFrame</Source><FeatureName></FeatureName></Origin><PrimaryAxis><DefinedDirection>+X</DefinedDirection><Source>ReferenceFrame</Source><SourceDirection>+Z</SourceDirection><FeatureName></FeatureName></PrimaryAxis><SecondaryAxis><DefinedDirection>+Y</DefinedDirection><Source>ReferenceFrame</Source><SourceDirection>+X</SourceDirection><FeatureName></FeatureName></SecondaryAxis></Value></Frame></Frames>  GraphicType=FromGeometry  MarkerShape=Sphere  MarkerSize=10  GraphicVisPropType=AdvancedVisualProperties  GraphicDiffuseColor="[0.2   0.2    0.2]"  GraphicSpecularColor="[0.8    0.8   0.8 1]"  GraphicAmbientColor=[0.05 0.05 0.05 1]  GraphicEmissiveColor=[0.0 0.0 0.0 1.0]  GraphicShininess=50  GraphicOpacity=1.0
  Rigid Transform : sm_lib/Frames and Transforms/Rigid Transform  TranslationMethod=Cartesian  TranslationStandardOffset=0  TranslationLengthUnit=m  TranslationStandardAxis=+Z  TranslationCartesianOffset=[0 -0.0015 0.0]  TranslationROffset=0  TranslationROffsetUnits=m  TranslationZOffset=0  TranslationZOffsetUnits=m  TranslationThetaOffset=0  TranslationThetaOffsetUnits=deg  RotationMethod=None  RotationAngleUnits=deg  RotationStandardAxis=+Z  RotationAngle=0.0  RotationArbitraryAxis=[0 0 1]  FollAlignAxisA=+X  BaseAlignAxisA=+Y  FollAlignAxisB=+Y  BaseAlignAxisB=+Z  RotationSequenceAxes=FollowerAxes  RotationSequence=XYX  RotationSequenceAngles=[0 0 0]  RotationSequenceAnglesUnits=deg  RotationMatrix=[1 0 0; 0 1 0; 0 0 1]
  Rigid Transform2 : sm_lib/Frames and Transforms/Rigid Transform  TranslationMethod=Cartesian  TranslationStandardOffset=1  TranslationLengthUnit=m  TranslationStandardAxis=+X  TranslationCartesianOffset=[-.075 -0.225 0]  TranslationROffset=0  TranslationROffsetUnits=m  TranslationZOffset=0  TranslationZOffsetUnits=m  TranslationThetaOffset=0  TranslationThetaOffsetUnits=deg  RotationMethod=None  RotationAngleUnits=deg  RotationStandardAxis=+Z  RotationAngle=0.0  RotationArbitraryAxis=[0 0 1]  FollAlignAxisA=+X  BaseAlignAxisA=+Y  FollAlignAxisB=+Y  BaseAlignAxisB=+Z  RotationSequenceAxes=FollowerAxes  RotationSequence=XYX  RotationSequenceAngles=[0 0 0]  RotationSequenceAnglesUnits=deg  RotationMatrix=[1 0 0; 0 1 0; 0 0 1]
  Rigid Transform3 : sm_lib/Frames and Transforms/Rigid Transform  TranslationMethod=StandardAxis  TranslationStandardOffset=0  TranslationLengthUnit=m  TranslationStandardAxis=+Y  TranslationCartesianOffset=[0 0 0]  TranslationROffset=0  TranslationROffsetUnits=m  TranslationZOffset=0  TranslationZOffsetUnits=m  TranslationThetaOffset=0  TranslationThetaOffsetUnits=deg  RotationMethod=StandardAxis  RotationAngleUnits=deg  RotationStandardAxis=+Y  RotationAngle=90  RotationArbitraryAxis=[0 0 1]  FollAlignAxisA=+X  BaseAlignAxisA=+Y  FollAlignAxisB=+Y  BaseAlignAxisB=+Z  RotationSequenceAxes=FollowerAxes  RotationSequence=XYX  RotationSequenceAngles=[0 0 0]  RotationSequenceAnglesUnits=deg  RotationMatrix=[1 0 0; 0 1 0; 0 0 1]
  Rigid Transform5 : sm_lib/Frames and Transforms/Rigid Transform  TranslationMethod=Cartesian  TranslationStandardOffset=1  TranslationLengthUnit=m  TranslationStandardAxis=+X  TranslationCartesianOffset=[0.075 -0.225 0]  TranslationROffset=0  TranslationROffsetUnits=m  TranslationZOffset=0  TranslationZOffsetUnits=m  TranslationThetaOffset=0  TranslationThetaOffsetUnits=deg  RotationMethod=None  RotationAngleUnits=deg  RotationStandardAxis=+Z  RotationAngle=0.0  RotationArbitraryAxis=[0 0 1]  FollAlignAxisA=+X  BaseAlignAxisA=+Y  FollAlignAxisB=+Y  BaseAlignAxisB=+Z  RotationSequenceAxes=FollowerAxes  RotationSequence=XYX  RotationSequenceAngles=[0 0 0]  RotationSequenceAnglesUnits=deg  RotationMatrix=[1 0 0; 0 1 0; 0 0 1]
  contact_ball+ : sm_lib/Body Elements/Spherical Solid  GraphicAmbientColor=[0.15 0.15 0.15 1.0]  BasedOnType=Density  CenterOfMass=[0 0 0]  CenterOfMassUnits=m  GraphicDiffuseColor="[ 0.9290    0.6940    0.1250]"  Density=1000  DensityUnits=kg/m^3  DoExposeReferenceFrame=on  GraphicEmissiveColor=[0.0 0.0 0.0 1.0]  ExportEntireGeometry=on  SerializedExposedGeometries=<ExposedGeometries><ExposedGeometry><RawGeometryId>entire</RawGeometryId><ExposedGeometryId>G</ExposedGeometryId></ExposedGeometry></ExposedGeometries>  SerializedFrames=<Frames/>  MarkerShape=Sphere  MarkerSize=10  GraphicType=FromGeometry  InertiaType=CalculateFromGeometry  Mass=1  MassUnits=kg  MomentsOfInertia=[1 1 1]  MomentsOfInertiaUnits=kg*m^2  GraphicOpacity=1.0  ProductsOfInertia=[0 0 0]  ProductsOfInertiaUnits=kg*m^2  GraphicShininess=75  GraphicSpecularColor=[0.5 0.5 0.5 1.0]  SphereRadius=0.0075  SphereRadiusUnits=m  GraphicVisPropType=SimpleVisualProperties
  contact_ball- : sm_lib/Body Elements/Spherical Solid  GraphicAmbientColor=[0.15 0.15 0.15 1.0]  BasedOnType=Density  CenterOfMass=[0 0 0]  CenterOfMassUnits=m  GraphicDiffuseColor="[ 0.9290    0.6940    0.1250]"  Density=1000  DensityUnits=kg/m^3  DoExposeReferenceFrame=on  GraphicEmissiveColor=[0.0 0.0 0.0 1.0]  ExportEntireGeometry=on  SerializedExposedGeometries=<ExposedGeometries><ExposedGeometry><RawGeometryId>entire</RawGeometryId><ExposedGeometryId>G</ExposedGeometryId></ExposedGeometry></ExposedGeometries>  SerializedFrames=<Frames/>  MarkerShape=Sphere  MarkerSize=10  GraphicType=FromGeometry  InertiaType=CalculateFromGeometry  Mass=1  MassUnits=kg  MomentsOfInertia=[1 1 1]  MomentsOfInertiaUnits=kg*m^2  GraphicOpacity=1.0  ProductsOfInertia=[0 0 0]  ProductsOfInertiaUnits=kg*m^2  GraphicShininess=75  GraphicSpecularColor=[0.5 0.5 0.5 1.0]  SphereRadius=0.0075  SphereRadiusUnits=m  GraphicVisPropType=SimpleVisualProperties
  W : PMIOPort  Side=Right
  Cart : PMIOPort  Port=2  Side=Right
  Rail : PMIOPort  Port=3  Side=Left
  connections:
  File Solid2/RConn1 -- Rigid Transform2/RConn1 -- Rigid Transform5/RConn1 -- Rigid Transform3/LConn1 -- Rigid Transform/LConn1
  contact_ball+/RConn1 -- Rigid Transform5/LConn1
  Rigid Transform3/RConn1 -- Rail/RConn1
  W/RConn1 -- Rigid Transform/RConn1
  Cart/RConn1 -- contact_ball+/LConn1
  contact_ball-/RConn1 -- Rigid Transform2/LConn1

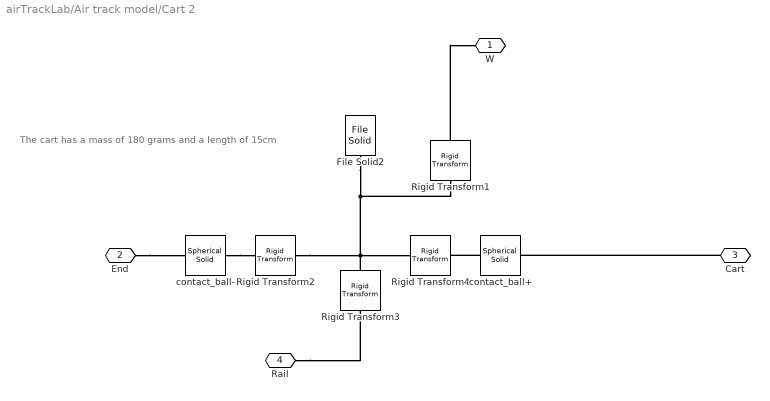
== system airTrackLab/Air track model/Cart 2 ==
  note: The cart has a mass of 180 grams and a length of 15cm
  File Solid2 : sm_lib/Body Elements/File Solid  ExtGeomFileName=cart.stl  UnitType=Custom  ExtGeomFileUnits=mm  StepReaderType=HEX  ExportConvexHullGeometry=off  InertiaType=PointMass  Mass=180  MassUnits=g  CenterOfMass=[0 0 0]  CenterOfMassUnits=m  MomentsOfInertia=[1 1 1]  MomentsOfInertiaUnits=kg*m^2  ProductsOfInertia=[0 0 0]  ProductsOfInertiaUnits=kg*m^2  BasedOnType=Density  Density=1000  DensityUnits=kg/m^3  DoExposeReferenceFrame=on  SerializedFrames=<Frames><Frame><Id>Frame1</Id><Value><Name>F1</Name><Origin><Source>CenterOfMassFrame</Source><FeatureName></FeatureName></Origin><PrimaryAxis><DefinedDirection>+X</DefinedDirection><Source>ReferenceFrame</Source><SourceDirection>+Z</SourceDirection><FeatureName></FeatureName></PrimaryAxis><SecondaryAxis><DefinedDirection>+Y</DefinedDirection><Source>ReferenceFrame</Source><SourceDirection>+X</SourceDirection><FeatureName></FeatureName></SecondaryAxis></Value></Frame></Frames>  GraphicType=FromGeometry  MarkerShape=Sphere  MarkerSize=10  GraphicVisPropType=AdvancedVisualProperties  GraphicDiffuseColor="[0.2   0.2    0.2]"  GraphicSpecularColor="[0.8    0.8   0.8 1]"  GraphicAmbientColor=[0.05 0.05 0.05 1]  GraphicEmissiveColor=[0.0 0.0 0.0 1.0]  GraphicShininess=50  GraphicOpacity=1.0
  Rigid Transform1 : sm_lib/Frames and Transforms/Rigid Transform  TranslationMethod=Cartesian  TranslationStandardOffset=0  TranslationLengthUnit=m  TranslationStandardAxis=+Z  TranslationCartesianOffset=[0 -0.0015 0.0]  TranslationROffset=0  TranslationROffsetUnits=m  TranslationZOffset=0  TranslationZOffsetUnits=m  TranslationThetaOffset=0  TranslationThetaOffsetUnits=deg  RotationMethod=None  RotationAngleUnits=deg  RotationStandardAxis=+Z  RotationAngle=0.0  RotationArbitraryAxis=[0 0 1]  FollAlignAxisA=+X  BaseAlignAxisA=+Y  FollAlignAxisB=+Y  BaseAlignAxisB=+Z  RotationSequenceAxes=FollowerAxes  RotationSequence=XYX  RotationSequenceAngles=[0 0 0]  RotationSequenceAnglesUnits=deg  RotationMatrix=[1 0 0; 0 1 0; 0 0 1]
  Rigid Transform2 : sm_lib/Frames and Transforms/Rigid Transform  TranslationMethod=Cartesian  TranslationStandardOffset=1  TranslationLengthUnit=m  TranslationStandardAxis=+X  TranslationCartesianOffset=[-.075 -0.225 0]  TranslationROffset=0  TranslationROffsetUnits=m  TranslationZOffset=0  TranslationZOffsetUnits=m  TranslationThetaOffset=0  TranslationThetaOffsetUnits=deg  RotationMethod=None  RotationAngleUnits=deg  RotationStandardAxis=+Z  RotationAngle=0.0  RotationArbitraryAxis=[0 0 1]  FollAlignAxisA=+X  BaseAlignAxisA=+Y  FollAlignAxisB=+Y  BaseAlignAxisB=+Z  RotationSequenceAxes=FollowerAxes  RotationSequence=XYX  RotationSequenceAngles=[0 0 0]  RotationSequenceAnglesUnits=deg  RotationMatrix=[1 0 0; 0 1 0; 0 0 1]
  Rigid Transform3 : sm_lib/Frames and Transforms/Rigid Transform  TranslationMethod=StandardAxis  TranslationStandardOffset=0  TranslationLengthUnit=m  TranslationStandardAxis=+Y  TranslationCartesianOffset=[0 0 0]  TranslationROffset=0  TranslationROffsetUnits=m  TranslationZOffset=0  TranslationZOffsetUnits=m  TranslationThetaOffset=0  TranslationThetaOffsetUnits=deg  RotationMethod=StandardAxis  RotationAngleUnits=deg  RotationStandardAxis=+Y  RotationAngle=90  RotationArbitraryAxis=[0 0 1]  FollAlignAxisA=+X  BaseAlignAxisA=+Y  FollAlignAxisB=+Y  BaseAlignAxisB=+Z  RotationSequenceAxes=FollowerAxes  RotationSequence=XYX  RotationSequenceAngles=[0 0 0]  RotationSequenceAnglesUnits=deg  RotationMatrix=[1 0 0; 0 1 0; 0 0 1]
  Rigid Transform4 : sm_lib/Frames and Transforms/Rigid Transform  TranslationMethod=Cartesian  TranslationStandardOffset=1  TranslationLengthUnit=m  TranslationStandardAxis=+X  TranslationCartesianOffset=[0.075 -0.225 0]  TranslationROffset=0  TranslationROffsetUnits=m  TranslationZOffset=0  TranslationZOffsetUnits=m  TranslationThetaOffset=0  TranslationThetaOffsetUnits=deg  RotationMethod=None  RotationAngleUnits=deg  RotationStandardAxis=+Z  RotationAngle=0.0  RotationArbitraryAxis=[0 0 1]  FollAlignAxisA=+X  BaseAlignAxisA=+Y  FollAlignAxisB=+Y  BaseAlignAxisB=+Z  RotationSequenceAxes=FollowerAxes  RotationSequence=XYX  RotationSequenceAngles=[0 0 0]  RotationSequenceAnglesUnits=deg  RotationMatrix=[1 0 0; 0 1 0; 0 0 1]
  contact_ball+ : sm_lib/Body Elements/Spherical Solid  GraphicAmbientColor=[0.15 0.15 0.15 1.0]  BasedOnType=Density  CenterOfMass=[0 0 0]  CenterOfMassUnits=m  GraphicDiffuseColor="[ 0.9290    0.6940    0.1250]"  Density=1000  DensityUnits=kg/m^3  DoExposeReferenceFrame=on  GraphicEmissiveColor=[0.0 0.0 0.0 1.0]  ExportEntireGeometry=on  SerializedExposedGeometries=<ExposedGeometries><ExposedGeometry><RawGeometryId>entire</RawGeometryId><ExposedGeometryId>G</ExposedGeometryId></ExposedGeometry></ExposedGeometries>  SerializedFrames=<Frames/>  MarkerShape=Sphere  MarkerSize=10  GraphicType=FromGeometry  InertiaType=CalculateFromGeometry  Mass=1  MassUnits=kg  MomentsOfInertia=[1 1 1]  MomentsOfInertiaUnits=kg*m^2  GraphicOpacity=1.0  ProductsOfInertia=[0 0 0]  ProductsOfInertiaUnits=kg*m^2  GraphicShininess=75  GraphicSpecularColor=[0.5 0.5 0.5 1.0]  SphereRadius=0.0075  SphereRadiusUnits=m  GraphicVisPropType=SimpleVisualProperties
  contact_ball- : sm_lib/Body Elements/Spherical Solid  GraphicAmbientColor=[0.15 0.15 0.15 1.0]  BasedOnType=Density  CenterOfMass=[0 0 0]  CenterOfMassUnits=m  GraphicDiffuseColor="[ 0.9290    0.6940    0.1250]"  Density=1000  DensityUnits=kg/m^3  DoExposeReferenceFrame=on  GraphicEmissiveColor=[0.0 0.0 0.0 1.0]  ExportEntireGeometry=on  SerializedExposedGeometries=<ExposedGeometries><ExposedGeometry><RawGeometryId>entire</RawGeometryId><ExposedGeometryId>G</ExposedGeometryId></ExposedGeometry></ExposedGeometries>  SerializedFrames=<Frames/>  MarkerShape=Sphere  MarkerSize=10  GraphicType=FromGeometry  InertiaType=CalculateFromGeometry  Mass=1  MassUnits=kg  MomentsOfInertia=[1 1 1]  MomentsOfInertiaUnits=kg*m^2  GraphicOpacity=1.0  ProductsOfInertia=[0 0 0]  ProductsOfInertiaUnits=kg*m^2  GraphicShininess=75  GraphicSpecularColor=[0.5 0.5 0.5 1.0]  SphereRadius=0.0075  SphereRadiusUnits=m  GraphicVisPropType=SimpleVisualProperties
  W : PMIOPort  Side=Left
  End : PMIOPort  Port=2  Side=Left
  Cart : PMIOPort  Port=3  Side=Right
  Rail : PMIOPort  Port=4  Side=Right
  connections:
  Rigid Transform1/RConn1 -- W/RConn1
  Rigid Transform3/LConn1 -- Rigid Transform1/LConn1 -- File Solid2/RConn1 -- Rigid Transform4/RConn1 -- Rigid Transform2/RConn1
  Cart/RConn1 -- contact_ball+/LConn1
  contact_ball+/RConn1 -- Rigid Transform4/LConn1
  contact_ball-/RConn1 -- Rigid Transform2/LConn1
  End/RConn1 -- contact_ball-/LConn1
  Rail/RConn1 -- Rigid Transform3/RConn1

== system airTrackLab/Air track model/Contact Force ==
  Elastic : Subsystem  VariantControl=Elastic
      mask Display: image('collisionElastic.png');
  Inelastic : Subsystem  VariantControl=Inelastic
      mask Display: image('collisionInelastic.png');
  G1 : PMIOPort  Side=Left
  G2 : PMIOPort  Port=2  Side=Right
  F1 : PMIOPort  Port=3  Side=Left
  F2 : PMIOPort  Port=4  Side=Right

== system airTrackLab/Air track model/Endstop L ==
  Contact Ball : sm_lib/Body Elements/Spherical Solid  GraphicAmbientColor=[0.15 0.15 0.15 1.0]  BasedOnType=Density  CenterOfMass=[0 0 0]  CenterOfMassUnits=m  GraphicDiffuseColor="[ 0.9290    0.6940    0.1250]"  Density=1000  DensityUnits=kg/m^3  DoExposeReferenceFrame=on  GraphicEmissiveColor=[0.0 0.0 0.0 1.0]  ExportEntireGeometry=off  SerializedExposedGeometries=<ExposedGeometries/>  SerializedFrames=<Frames/>  MarkerShape=Sphere  MarkerSize=10  GraphicType=FromGeometry  InertiaType=CalculateFromGeometry  Mass=1  MassUnits=kg  MomentsOfInertia=[1 1 1]  MomentsOfInertiaUnits=kg*m^2  GraphicOpacity=1.0  ProductsOfInertia=[0 0 0]  ProductsOfInertiaUnits=kg*m^2  GraphicShininess=75  GraphicSpecularColor=[0.5 0.5 0.5 1.0]  SphereRadius=0.0075  SphereRadiusUnits=m  GraphicVisPropType=SimpleVisualProperties
  Endstop : sm_lib/Body Elements/File Solid  ExtGeomFileName=stop.stl  UnitType=Custom  ExtGeomFileUnits=mm  StepReaderType=HEX  ExportConvexHullGeometry=off  InertiaType=PointMass  Mass=180  MassUnits=g  CenterOfMass=[0 0 0]  CenterOfMassUnits=m  MomentsOfInertia=[1 1 1]  MomentsOfInertiaUnits=kg*m^2  ProductsOfInertia=[0 0 0]  ProductsOfInertiaUnits=kg*m^2  BasedOnType=Density  Density=1000  DensityUnits=kg/m^3  DoExposeReferenceFrame=on  SerializedFrames=<Frames/>  GraphicType=FromGeometry  MarkerShape=Sphere  MarkerSize=10  GraphicVisPropType=AdvancedVisualProperties  GraphicDiffuseColor="[0.2   0.2    0.2]"  GraphicSpecularColor="[0.8    0.8   0.8 1]"  GraphicAmbientColor=[0.05 0.05 0.05 1]  GraphicEmissiveColor=[0.0 0.0 0.0 1.0]  GraphicShininess=50  GraphicOpacity=1.0
  Rigid Transform1 : sm_lib/Frames and Transforms/Rigid Transform  TranslationMethod=Cartesian  TranslationStandardOffset=1  TranslationLengthUnit=m  TranslationStandardAxis=+X  TranslationCartesianOffset=[1-0.003 -0.225 0]  TranslationROffset=0  TranslationROffsetUnits=m  TranslationZOffset=0  TranslationZOffsetUnits=m  TranslationThetaOffset=0  TranslationThetaOffsetUnits=deg  RotationMethod=None  RotationAngleUnits=deg  RotationStandardAxis=+Z  RotationAngle=0.0  RotationArbitraryAxis=[0 0 1]  FollAlignAxisA=+X  BaseAlignAxisA=+Y  FollAlignAxisB=+Y  BaseAlignAxisB=+Z  RotationSequenceAxes=FollowerAxes  RotationSequence=XYX  RotationSequenceAngles=[0 0 0]  RotationSequenceAnglesUnits=deg  RotationMatrix=[1 0 0; 0 1 0; 0 0 1]
  R : PMIOPort  Side=Right
  connections:
  Endstop/RConn1 -- Rigid Transform1/RConn1 -- R/RConn1
  Contact Ball/RConn1 -- Rigid Transform1/LConn1
